simulink model "riduzione_stato"  (R2023b)
settings: Solver=FixedStepAuto  StartTime=0.0  StopTime=inf  RelTol=1e-3  EnableMultiTasking=on
undefined symbols (not defined in the file): K, Ki, Ts
libraries: mbedblockslib x3, stm_qeplib x1
settings Model: ExtModeTrigDuration=10  Creator=acoon  LastModifiedBy=Beniamino
settings OptimizationCC: EnhancedBackFolding=on  PassReuseOutputArgsThreshold=0  MaxStackSize=64  OptimizeBlockOrder=speed  DifferentSizesBufferReuse=on  OptimizationCustomize=off
settings DebuggingCC: ParameterTunabilityLossMsg=error
settings HardwareCC: ProdBitPerPointer=32  ProdBitPerSizeT=32  ProdBitPerPtrDiffT=32  ProdLargestAtomicInteger=Long  ProdLargestAtomicFloat=Double  ProdWordSize=32  ProdLongLongMode=on  ProdHWDeviceType=ARM Compatible->ARM Cortex  UseEmbeddedCoderFeatures=off
settings SFSimCC: MATLABDynamicMemAlloc=off
settings RTWCC: Description=Embedded Coder  SystemTargetFile=ert.tlc  HardwareBoard=STM32 Nucleo F401RE  TemplateMakefile=ert_default_tmf  Toolchain=GNU Tools for ARM Embedded Processors
settings CodeAppCC: ForceParamTrailComments=on  OperatorAnnotations=on
settings ERTTargetCC: ERTCustomFileBanners=off  SupportContinuousTime=on  SupportNonInlinedSFcns=on  RemoveResetFunc=off  ModelStepFunctionPrototypeControlCompliant=off  ExtModeTransport=3  ExtModeStaticAlloc=on  ExtModeStaticAllocSize=2000  ExtModeMexFile=ext_xcp  ExtModeIntrfLevel=Level2 - Open

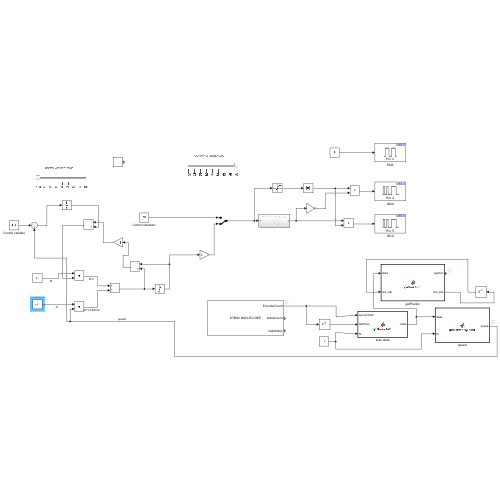
[thumbnail: Simulink's stored preview of the top-level diagram]
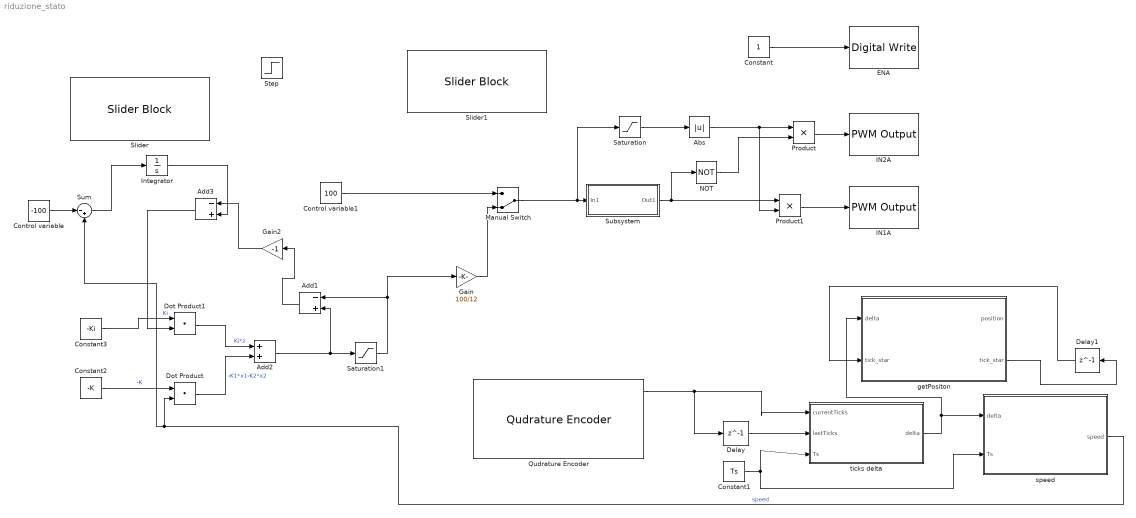
== system riduzione_stato ==
  Abs : Abs  SaturateOnIntegerOverflow=off
  Add1 : Sum  Inputs=-+
  Add2 : Sum
  Add3 : Sum  Inputs=-+
  Constant : Constant
  Constant1 : Constant  Value=Ts
  Constant2 : Constant  Value=-K
  Constant3 : Constant  Value=-Ki
  Control variable : Constant  Value=-100
  Control variable1 : Constant  Value=100
  Delay : Delay  DelayLength=1
  Delay1 : Delay  DelayLength=1  InitialCondition=0
  Dot Product : DotProduct  OutDataTypeStr=Inherit: Inherit via internal rule
  Dot Product1 : DotProduct  OutDataTypeStr=Inherit: Inherit via internal rule
  ENA : mbedblockslib/Digital Write  Pin=2  Direction=output
      settings: LibrarySourceBlock=stmnucleorootlib/Common/Digital Write
  Gain : Gain  Gain=100/12
  Gain2 : Gain  Gain=-1
  IN1A : mbedblockslib/PWM Output  Pin=5  EnableInputFrequency=off  InitialFrequency=2000  InitialDutyCycle=50  NotificationType=None
      settings: LibrarySourceBlock=stmnucleorootlib/Common/PWM Output
  IN2A : mbedblockslib/PWM Output  Pin=4  EnableInputFrequency=off  InitialFrequency=2000  InitialDutyCycle=50  NotificationType=None
      settings: LibrarySourceBlock=stmnucleorootlib/Common/PWM Output
  Integrator : Integrator
  Manual Switch : ManualSwitch  CurrentSetting=0
  NOT : Logic  Operator=NOT  IconShape=distinctive  AllPortsSameDT=off  OutDataTypeStr=boolean
  Product : Product
  Product1 : Product
  Qudrature Encoder : stm_qeplib/Qudrature Encoder  SampleTime=Ts
  Saturation : Saturate  UpperLimit=100  LowerLimit=-100
  Saturation1 : Saturate  UpperLimit=12  LowerLimit=-12
  Slider : SliderBlock  ScaleMin=-100
  Slider1 : SliderBlock  ScaleMin=-100
  Step : Step  After=50  SampleTime=0
  Subsystem : Subsystem
  Sum : Sum  Inputs=|-+
  getPositon : MATLAB Function  TreatAsAtomicUnit=on
  speed : MATLAB Function  TreatAsAtomicUnit=on
  ticks delta : MATLAB Function  TreatAsAtomicUnit=on
  wires:
  Constant/1 -> ENA/1
  Product/1 -> IN2A/1
  Product1/1 -> IN1A/1
  Saturation/1 -> Abs/1
  Abs/1 -> Product/1, Product1/2
  NOT/1 -> Product/2
  Subsystem/1(Out1) -> Product1/1, NOT/1
  ticks delta/1(delta) -> getPositon/1(delta), speed/1(delta)
  Delay/1 -> ticks delta/2(lastTicks)
  Qudrature Encoder/1 -> ticks delta/1(currentTicks), Delay/1
  Constant1/1 -> ticks delta/3(Ts), speed/2(Ts)
  getPositon/2(tick_star) -> Delay1/1
  Delay1/1 -> getPositon/2("tick_star ")
  Control variable/1 -> Sum/1
  Constant3/1 -> Dot Product1/1  "Ki"
  Dot Product1/1 -> Add2/1  "Ki*z"
  Dot Product/1 -> Add2/2  "-K1*x1-K2*x2"
  Constant2/1 -> Dot Product/1  "-K"
  speed/1(speed) -> Sum/2, Dot Product/2  "speed"
  Manual Switch/1 -> Saturation/1, Subsystem/1(In1)
  Control variable1/1 -> Manual Switch/1
  Add2/1 -> Add1/2, Saturation1/1
  Saturation1/1 -> Gain/1, Add1/1
  Gain/1 -> Manual Switch/2
  Add1/1 -> Gain2/1
  Gain2/1 -> Add3/1
  Sum/1 -> Integrator/1
  Integrator/1 -> Add3/2
  Add3/1 -> Dot Product1/2

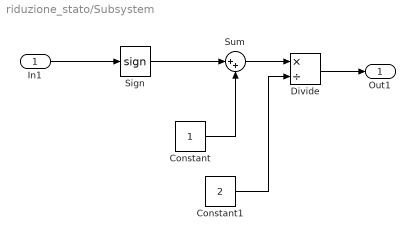
== system riduzione_stato/Subsystem ==
  In1 : Inport
  Constant : Constant
  Constant1 : Constant  Value=2
  Divide : Product  Inputs=*/
  Sign : Signum
  Sum : Sum  Inputs=|++
  Out1 : Outport
  wires:
  In1/1 -> Sign/1
  Sign/1 -> Sum/1
  Constant/1 -> Sum/2
  Sum/1 -> Divide/1
  Divide/1 -> Out1/1
  Constant1/1 -> Divide/2

== matlab function riduzione_stato/ticks delta ==
  data: currentTicks input; lastTicks input; delta output; Ts input
function delta = getTicksData(currentTicks, lastTicks, Ts)

currentTicks = double(currentTicks);
lastTicks = double(lastTicks);

if abs(currentTicks - lastTicks) <= ceil(12600*Ts)
    delta = currentTicks - lastTicks;
else
    if lastTicks > currentTicks
        delta = currentTicks + 2^16-1 - lastTicks;
    else
        delta = currentTicks - 2^16+1 - lastTicks;
    end
end

end

== matlab function riduzione_stato/getPositon ==
  data: delta input; position output; tick_star input; tick_star output
function [position, tick_star] = getPosition(delta, tick_star)

tick_star = double(tick_star + delta);

completeTheta = 2 * pi * tick_star /(8400);

position = sign(completeTheta) * mod(abs(completeTheta), 2*pi);

end

== matlab function riduzione_stato/speed ==
  data: delta input; speed output; Ts input
function speed = getSpeedByDelta(delta, Ts)

speed = delta * 60 / (8400*Ts);

end
